simulink subsystem "Pump"  (R2024b)
settings: Solver=VariableStepAuto  StartTime=0.0  StopTime=10.0  RelTol=1e-3
undefined symbols (not defined in the file or in its folder): pump
libraries: fl_lib x16, nesl_utility x4, SimscapeFluids_lib x1
settings Model: Creator=saprasad  LastModifiedBy=jjha
settings RTWCC: GPUComputeCapability=3.5

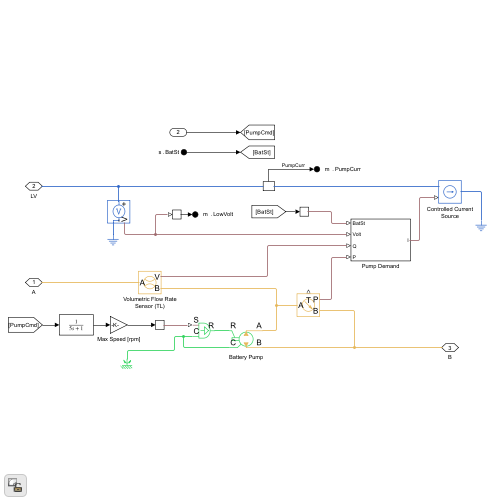
[thumbnail: Simulink's stored preview of the top-level diagram]
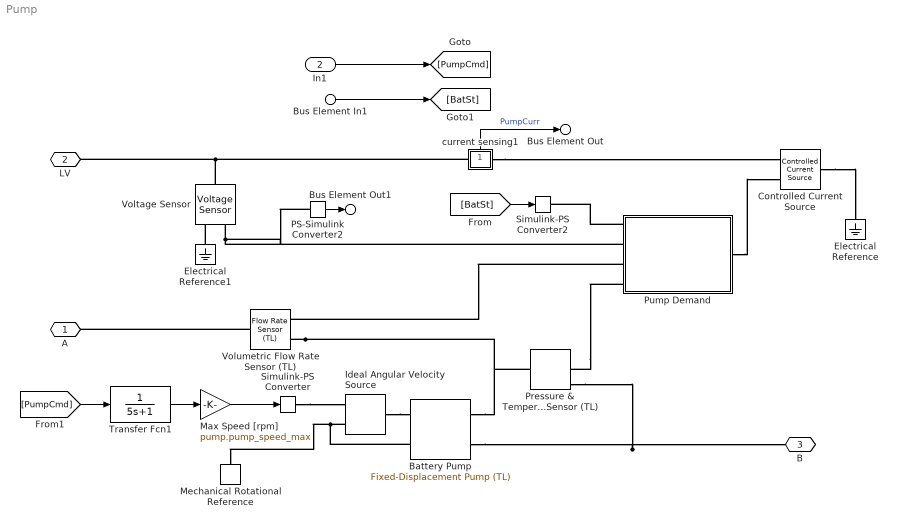
== system Pump ==
  Bus Element In1 : Inport  PortName=s  Element=BatSt
  In1 : Inport  Port=2
  Battery Pump : SimscapeFluids_lib/Thermal Liquid/Pumps & Motors/Fixed-Displacement Pump (TL)  loss_spec=1  displacement=pump.pump_displacement l/rev  omega_nominal=0.5 * pump.pump_speed_max rpm  p_nominal=0.1 MPa  mu_nominal=0.9 cP  vol_eff_nominal=0.92  mech_eff_nominal=1/(1 + (0.6)/(pump.pump_displacement)*0.006283185307179586 + (0.05)/(pump.pump_displacement)/(0.1)*0.006283185307179586)  no_load_torque=0.05 N*m  p_diff_eff_TLU=[.1, 1, 2] MPa  omega_eff_TLU=[25, 50, 100, 200, 300, 400] rad/s  vol_eff_TLU=[.816, .908, .954, .977, .981, .984; .325, .663, .831, .916, .925, .946; .137, .568, .78, .892, .893, .91]  mech_eff_TLU=[.996, .996, .996, .996, .996, .996; .988, .989, .989, .989, .989, .99; .981, .981, .982, .982, .983, .984]  p_diff_loss_TLU=[.1, 1, 2] MPa  omega_loss_TLU=[25, 50, 100, 200, 300, 400] rad/s  vol_loss_TLU=[.023, .023, .023, .023, .0285, .032; .0844, .0842, .0845, .084, .1125, .108; .1079, .108, .11, .108, .1605, .18] * 1e-3 m^3/s  mech_loss_TLU=[.002, .002, .002, .002, .002, .002; .0607, .0556, .0556, .0556, .0556, .0505; .1937, .1937, .1833, .1833, .1729, .1626] N*m  vol_eff_min=1e-3  vol_eff_max=1  mech_eff_min=1e-3  mech_eff_max=1  pressure_threshold=1e-3 MPa  omega_threshold=10 rad/s  area=pi * pump.coolant_pipe_D^2 / 4 m^2  supplied_range_check=0  pump_mode_check=simscape.enum.assert.action.none  pressure_check=simscape.enum.assert.action.none  p_min_valid=0.101325 MPa
  Controlled Current Source : fl_lib/Electrical/Electrical Sources/Controlled Current Source
  Electrical Reference : fl_lib/Electrical/Electrical Elements/Electrical Reference
  Electrical Reference1 : fl_lib/Electrical/Electrical Elements/Electrical Reference
  Ideal Angular Velocity Source : fl_lib/Mechanical/Mechanical Sources/Ideal Angular Velocity Source
  Max Speed [rpm] : Gain  Gain=pump.pump_speed_max
  Mechanical Rotational Reference : fl_lib/Mechanical/Rotational Elements/Mechanical Rotational Reference
  PS-Simulink Converter2 : nesl_utility/PS-Simulink Converter  PhysicalDomain=network_engine_domain  SubClassName=ps_output  LeftPortType=input  RightPortType=output  PseudoPeriodic=off  Frequencies=[]  VectorFormat=inherit  Unit=inherit  AffineConversion=off
  Pressure & Temperature Sensor (TL) : fl_lib/Thermal Liquid/Sensors/Pressure & Temperature Sensor (TL)  reference=foundation.enum.MeasurementReference.difference  pressure=true  pressure_spec=foundation.enum.PressureMeasementSpec.Absolute  temperature=true
      settings: InternalSimscapePortConfiguration="{\"Bottom\":[{\"id\":\"T\",\"label\":\"T\",\"type\":\"output\"}],\"Left\":[{\"id\":\"A\",\"label\":\"A\",\"type\":\"foundation.thermal_liquid.thermal_liquid\"}],\"Right\":[{\"id\":\"B\",\"label\":\"B\",\"type\":\"foundation.thermal_liquid.thermal_liquid\"},{\"id\":\"P\",\"label\":\"P\",\"type\":\"output\"}],\"Top\":[]}"
  Pump Demand : Subsystem
  Simulink-PS Converter : nesl_utility/Simulink-PS Converter  PhysicalDomain=network_engine_domain  SubClassName=ps_input  LeftPortType=input  RightPortType=output  PseudoPeriodic=off  Frequencies=[]  NoiseDistribution=none  NoiseParameters=[]  Unit=rpm  AffineConversion=off  FilteringAndDerivatives=provide  SimscapeFilterOrder=1  InputFilterTimeConstant=0.001  UdotUserProvided=0
  Simulink-PS Converter2 : nesl_utility/Simulink-PS Converter  PhysicalDomain=network_engine_domain  SubClassName=ps_input  LeftPortType=input  RightPortType=output  PseudoPeriodic=off  Frequencies=[]  NoiseDistribution=none  NoiseParameters=[]  Unit=1  AffineConversion=off  FilteringAndDerivatives=provide  SimscapeFilterOrder=1  InputFilterTimeConstant=0.001  UdotUserProvided=0
  Transfer Fcn1 : TransferFcn  Denominator=[5 1]
  Voltage Sensor : fl_lib/Electrical/Electrical Sensors/Voltage Sensor
  Volumetric Flow Rate Sensor (TL) : fl_lib/Thermal Liquid/Sensors/Flow Rate Sensor (TL)  mass_flow_measure=false  volumetric_flow_measure=true  energy_flow_measure=false
      settings: InternalSimscapePortConfiguration="{\"Bottom\":[],\"Left\":[{\"id\":\"A\",\"label\":\"A\",\"type\":\"foundation.thermal_liquid.thermal_liquid\"}],\"Right\":[{\"id\":\"B\",\"label\":\"B\",\"type\":\"foundation.thermal_liquid.thermal_liquid\"},{\"id\":\"V\",\"label\":\"V\",\"type\":\"output\"}],\"Top\":[]}"
  current sensing1 : Subsystem
      settings: PortSchema="{\"entries\":[{\"content\":{\"sides\":[{\"content\":{\"connectorIds\":[\"LConn1\"]},\"type\":\"ConnectorPlacement.EquallySpacedRectSide\",\"uuid\":\"be2815b5-7c4b-4452-9f46-9765620d338b\"},{\"content\":{\"connectorIds\":[\"RConn1\"],\"side\":\"RIGHT\"},\"type\":\"ConnectorPlacement.EquallySpacedRectSide\",\"uuid\":\"398ebab2-f4fa-4d00-bf6e-74bf1f6972c5\"},{\"content\":{\"connectorIds\":[\"Out1\"],\"side\":\"TOP\"},\"type\":\"ConnectorPlacement.EquallySpacedRectSide\",\"uuid\":\"f18d5713-17ec-4be9-9072-3e03c5a4f599\"}]},\"type\":\"ConnectorPlacement.EquallySpacedConnector\",\"uuid\":\"966ec05e-6316-4039-8e26-1d6b096cf423\"}],\"packageUris\":[\"http://schema.mathworks.com/mf0/Connector/R2020b\"],\"version\":\"1.0\"}"
  A : PMIOPort  Side=Left
  LV : PMIOPort  Port=2  Side=Left
  B : PMIOPort  Port=3  Side=Right
  Bus Element Out : Outport  PortName=m  Element=PumpCurr
  Bus Element Out1 : Outport  PortName=m  Element=LowVolt
  wires:
  Bus Element In1/1 -> [BatSt]
  In1/1 -> [PumpCmd]
  [BatSt] -> Simulink-PS Converter2/1
  Transfer Fcn1/1 -> Max Speed [rpm]/1
  Max Speed [rpm]/1 -> Simulink-PS Converter/1
  [PumpCmd] -> Transfer Fcn1/1
  current sensing1/1("   ") -> Bus Element Out/1  "PumpCurr"
  PS-Simulink Converter2/1 -> Bus Element Out1/1
  connections:
  Voltage Sensor/LConn1 -- LV/RConn1 -- current sensing1/LConn1
  Ideal Angular Velocity Source/RConn2 -- Battery Pump/RConn2 -- Mechanical Rotational Reference/LConn1
  Pressure & Temperature Sensor (TL)/RConn1 -- B/RConn1 -- Battery Pump/LConn2
  Volumetric Flow Rate Sensor (TL)/RConn1 -- Pressure & Temperature Sensor (TL)/LConn1 -- Battery Pump/LConn1
  Voltage Sensor/RConn1 -- Pump Demand/LConn2 -- PS-Simulink Converter2/LConn1
  Pump Demand/LConn3 -- Volumetric Flow Rate Sensor (TL)/RConn2
  Pump Demand/LConn4 -- Pressure & Temperature Sensor (TL)/RConn2
  Controlled Current Source/LConn1 -- Electrical Reference/LConn1
  Pump Demand/RConn1 -- Controlled Current Source/RConn1
  Pump Demand/LConn1 -- Simulink-PS Converter2/RConn1
  Electrical Reference1/LConn1 -- Voltage Sensor/RConn2
  current sensing1/RConn1 -- Controlled Current Source/RConn2
  Volumetric Flow Rate Sensor (TL)/LConn1 -- A/RConn1
  Ideal Angular Velocity Source/LConn1 -- Battery Pump/RConn1
  Simulink-PS Converter/RConn1 -- Ideal Angular Velocity Source/RConn1

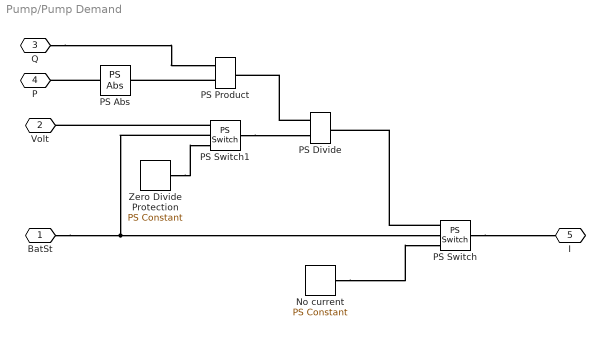
== system Pump/Pump Demand ==
  No current : fl_lib/Physical Signals/Sources/PS Constant  constant=0 A
  PS Abs : fl_lib/Physical Signals/Nonlinear Operators/PS Abs
      settings: InternalSimscapePortConfiguration="{\"Bottom\":[],\"Left\":[{\"id\":\"I\",\"label\":\"\",\"type\":\"input\"}],\"Right\":[{\"id\":\"O\",\"label\":\"\",\"type\":\"output\"}],\"Top\":[]}"
  PS Divide : fl_lib/Physical Signals/Functions/PS Divide
  PS Product : fl_lib/Physical Signals/Functions/PS Product
  PS Switch : fl_lib/Physical Signals/Nonlinear Operators/PS Switch  Threshold=0.5
      settings: InternalSimscapePortConfiguration="{\"Bottom\":[],\"Left\":[{\"id\":\"I1\",\"label\":\"\",\"type\":\"input\"},{\"id\":\"I2\",\"label\":\"\",\"type\":\"input\"},{\"id\":\"I3\",\"label\":\"\",\"type\":\"input\"}],\"Right\":[{\"id\":\"O\",\"label\":\"\",\"type\":\"output\"}],\"Top\":[]}"
  PS Switch1 : fl_lib/Physical Signals/Nonlinear Operators/PS Switch  Threshold=0.5
      settings: InternalSimscapePortConfiguration="{\"Bottom\":[],\"Left\":[{\"id\":\"I1\",\"label\":\"\",\"type\":\"input\"},{\"id\":\"I2\",\"label\":\"\",\"type\":\"input\"},{\"id\":\"I3\",\"label\":\"\",\"type\":\"input\"}],\"Right\":[{\"id\":\"O\",\"label\":\"\",\"type\":\"output\"}],\"Top\":[]}"
  Zero Divide Protection : fl_lib/Physical Signals/Sources/PS Constant  constant=1 V
  BatSt : PMIOPort  Side=Left
  Volt : PMIOPort  Port=2  Side=Left
  Q : PMIOPort  Port=3  Side=Left
  P : PMIOPort  Port=4  Side=Left
  I : PMIOPort  Port=5  Side=Right
  connections:
  No current/RConn1 -- PS Switch/LConn3
  PS Switch1/LConn1 -- Volt/RConn1
  PS Switch/LConn1 -- PS Divide/RConn1
  BatSt/RConn1 -- PS Switch/LConn2 -- PS Switch1/LConn2
  PS Switch/RConn1 -- I/RConn1
  PS Divide/LConn1 -- PS Product/RConn1
  Q/RConn1 -- PS Product/LConn1
  PS Abs/LConn1 -- P/RConn1
  PS Switch1/RConn1 -- PS Divide/LConn2
  Zero Divide Protection/RConn1 -- PS Switch1/LConn3
  PS Product/LConn2 -- PS Abs/RConn1

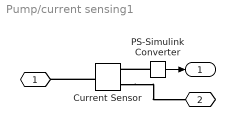
== system Pump/current sensing1 ==
  Current Sensor : fl_lib/Electrical/Electrical Sensors/Current Sensor
  PS-Simulink Converter : nesl_utility/PS-Simulink Converter  PhysicalDomain=network_engine_domain  SubClassName=ps_output  LeftPortType=input  RightPortType=output  PseudoPeriodic=off  Frequencies=[]  VectorFormat=inherit  Unit=inherit  AffineConversion=off
  "  " : PMIOPort  Side=Left
  " " : PMIOPort  Port=2  Side=Right
  "   " : Outport
  wires:
  PS-Simulink Converter/1 -> "   "/1
  connections:
  PS-Simulink Converter/LConn1 -- Current Sensor/RConn1
  Current Sensor/LConn1 -- "  "/RConn1
  Current Sensor/RConn2 -- " "/RConn1
